simulink model "Parcial3_validacion_datos"  (R2016a)
settings: Solver=VariableStepAuto  StartTime=0.0  StopTime=1500  RelTol=1e-3
values from neighbouring files (symbols this model uses):
  tm = 0.1    [ejemplodiscretro.m]
undefined symbols (not defined in the file or in its folder): anfisfuzzy, ts
libraries: fuzblock x1, simulink x1
settings Model: Creator=Daniel  LastModifiedBy=Daniel

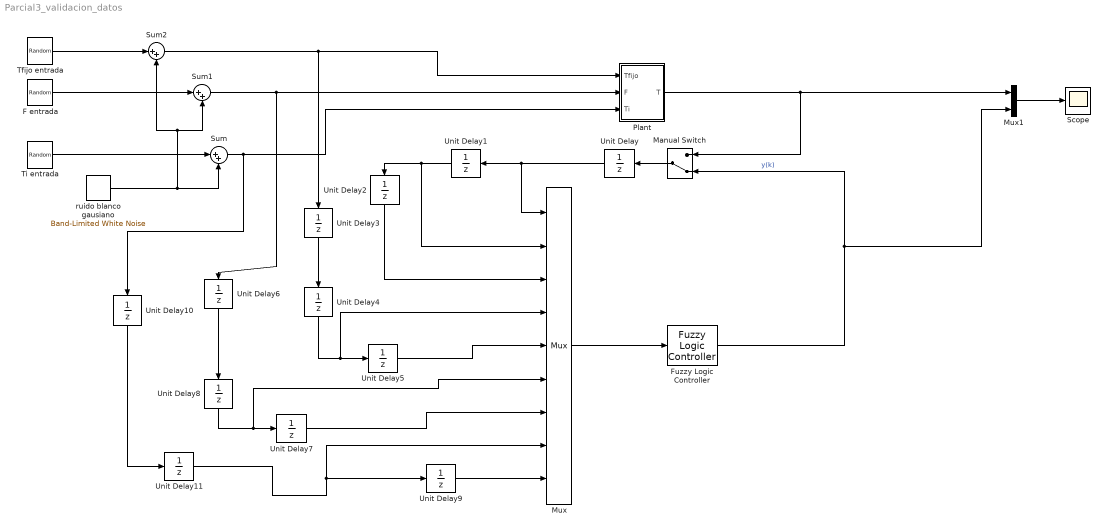
== system Parcial3_validacion_datos ==
  F entrada : UniformRandomNumber  Minimum=-4  Maximum=107  SampleTime=ts
  Fuzzy Logic Controller : fuzblock/Fuzzy Logic  Controller  fis=[anfisfuzzy]
  Manual Switch : ManualSwitch  CurrentSetting=0
  Mux : Mux  Inputs=9
  Mux1 : Mux  Inputs=2
  Plant : Subsystem
  Scope : Scope
  Sum : Sum  Inputs=|++
  Sum1 : Sum  Inputs=|++
  Sum2 : Sum  Inputs=|++
  Tfijo entrada : UniformRandomNumber  Minimum=-15  Maximum=270  SampleTime=ts
  Ti entrada : UniformRandomNumber  Minimum=-100  Maximum=320  SampleTime=ts
  Unit Delay{,1..11} (12 alike) : UnitDelay  SampleTime=tm
  ruido blanco gausiano : simulink/Sources/Band-Limited White Noise  Cov=[0.5]  Ts=tm  seed=[23341]
  wires:
  Fuzzy Logic Controller/1 -> Manual Switch/2, Mux1/2  "y(k)"
  Manual Switch/1 -> Unit Delay/1
  Mux1/1 -> Scope/1
  Mux/1 -> Fuzzy Logic Controller/1
  Plant/1(T) -> Manual Switch/1, Mux1/1
  F entrada/1 -> Sum1/1
  ruido blanco gausiano/1 -> Sum/2, Sum1/2, Sum2/2
  Tfijo entrada/1 -> Sum2/1
  Ti entrada/1 -> Sum/1
  Sum1/1 -> Plant/2(F), Unit Delay6/1
  Sum2/1 -> Unit Delay3/1, Plant/1(Tfijo)
  Sum/1 -> Plant/3(Ti), Unit Delay10/1
  Unit Delay/1 -> Mux/1, Unit Delay1/1
  Unit Delay1/1 -> Mux/2, Unit Delay2/1
  Unit Delay2/1 -> Mux/3
  Unit Delay3/1 -> Unit Delay4/1
  Unit Delay4/1 -> Mux/4, Unit Delay5/1
  Unit Delay5/1 -> Mux/5
  Unit Delay6/1 -> Unit Delay8/1
  Unit Delay8/1 -> Mux/6, Unit Delay7/1
  Unit Delay7/1 -> Mux/7
  Unit Delay10/1 -> Unit Delay11/1
  Unit Delay11/1 -> Mux/8, Unit Delay9/1
  Unit Delay9/1 -> Mux/9

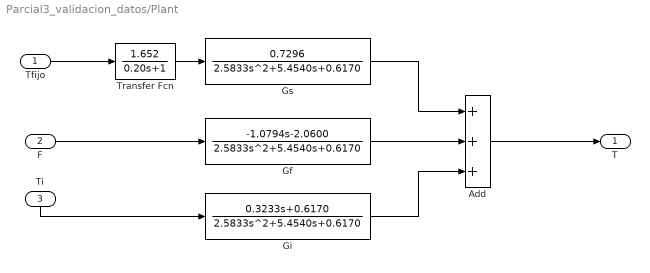
== system Parcial3_validacion_datos/Plant ==
  Tfijo : Inport
  F : Inport  Port=2
  Ti : Inport  Port=3
  Add : Sum  Inputs=+++
  Gf : TransferFcn  Numerator=[-1.0794 -2.0600]  Denominator=[2.5833 5.4540 0.6170]
  Gi : TransferFcn  Numerator=[0.3233 0.6170]  Denominator="[2.5833 5.4540  0.6170]"
  Gs : TransferFcn  Numerator=[0.7296]  Denominator="[2.5833 5.4540  0.6170]"
  Transfer Fcn : TransferFcn  Numerator=[1.652]  Denominator=[0.20 1]
  T : Outport
  wires:
  Add/1 -> T/1
  Gi/1 -> Add/3
  Gf/1 -> Add/2
  Transfer Fcn/1 -> Gs/1
  Gs/1 -> Add/1
  Ti/1 -> Gi/1
  Tfijo/1 -> Transfer Fcn/1
  F/1 -> Gf/1
